simulink library "INT_GlbDa_SetData"  (R2016b)
settings: Solver=VariableStepAuto  StartTime=0.0  StopTime=10.0  RelTol=1e-3
settings Model: Creator=Administrator  LastModifiedBy=Administrator

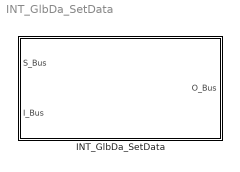
== system INT_GlbDa_SetData ==
  INT_GlbDa_SetData : Subsystem

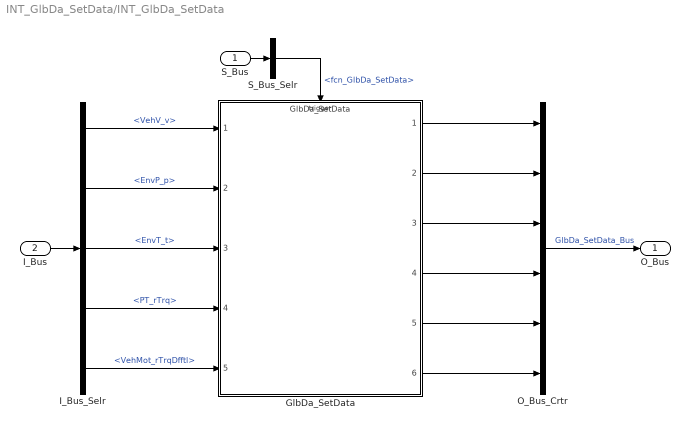
== system INT_GlbDa_SetData/INT_GlbDa_SetData ==
  S_Bus : Inport
  I_Bus : Inport  Port=2
  GlbDa_SetData : ModelReference  ModelNameDialog=GlbDa_SetData  SimulationMode=Normal  ModelReferenceVersion=1.10  TriggerPortName=function  TriggerPortTriggerType=function-call  TriggerPortStatesWhenEnabling=held
  I_Bus_Selr : BusSelector  OutputSignals=VehV_v,EnvP_p,EnvT_t,PT_rTrq,VehMot_rTrqDfftl
  O_Bus_Crtr : BusCreator  Inputs=6
  S_Bus_Selr : BusSelector  OutputSignals=fcn_GlbDa_SetData
  O_Bus : Outport
  wires:
  S_Bus_Selr/1 -> GlbDa_SetData/Trigger  "<fcn_GlbDa_SetData>"
  S_Bus/1 -> S_Bus_Selr/1
  I_Bus/1 -> I_Bus_Selr/1
  I_Bus_Selr/1 -> GlbDa_SetData/1  "<VehV_v>"
  I_Bus_Selr/2 -> GlbDa_SetData/2  "<EnvP_p>"
  I_Bus_Selr/3 -> GlbDa_SetData/3  "<EnvT_t>"
  I_Bus_Selr/4 -> GlbDa_SetData/4  "<PT_rTrq>"
  I_Bus_Selr/5 -> GlbDa_SetData/5  "<VehMot_rTrqDfftl>"
  O_Bus_Crtr/1 -> O_Bus/1  "GlbDa_SetData_Bus"
  GlbDa_SetData/1 -> O_Bus_Crtr/1
  GlbDa_SetData/2 -> O_Bus_Crtr/2
  GlbDa_SetData/3 -> O_Bus_Crtr/3
  GlbDa_SetData/4 -> O_Bus_Crtr/4
  GlbDa_SetData/5 -> O_Bus_Crtr/5
  GlbDa_SetData/6 -> O_Bus_Crtr/6
